simulink model "essrampa"  (R2014a)
settings: Solver=ode45  StartTime=0.0  StopTime=100  RelTol=1e-3
libraries: simulink x1
settings Model: Creator=Nury  LastModifiedBy=Nury
settings DebuggingCC: SolverPrmCheckMsg=none

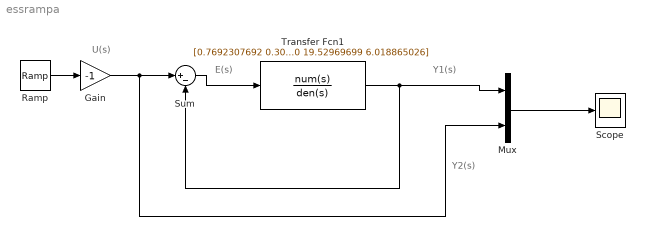
== system essrampa ==
  note: Y2(s)
  note: Y1(s)
  note: E(s)
  note: U(s)
  Gain : Gain  Gain=-1
  Mux : Mux  Inputs=2
  Ramp : simulink/Sources/Ramp  slope=1  start=0  X0=0
  Scope : Scope
      settings: YMin=5000  YMax=32500
  Sum : Sum  Inputs=|+-
  Transfer Fcn1 : TransferFcn  Numerator=[0.7692307692 0.3076923077 15.02284384]  Denominator=[1 0.40 19.52969699 6.018865026]
  wires:
  Gain/1 -> Mux/2, Sum/1
  Sum/1 -> Transfer Fcn1/1
  Mux/1 -> Scope/1
  Transfer Fcn1/1 -> Mux/1, Sum/2
  Ramp/1 -> Gain/1
